simulink subsystem "Corrections"  (R2023b)
settings: Solver=VariableStepAuto  StartTime=0.0  StopTime=10.0  RelTol=1e-3
values from neighbouring files (symbols this model uses):
  c = obj.body_coeffs.Cnm.value    [SH_nav.m]
undefined symbols (not defined in the file or in its folder): Propagation, R_st, v_b, v_m, x_b, x_m
libraries: nav_lib x10, simulink x2, matrix_library x2, vrlib x1
settings Model: Creator=brent  LastModifiedBy=brent

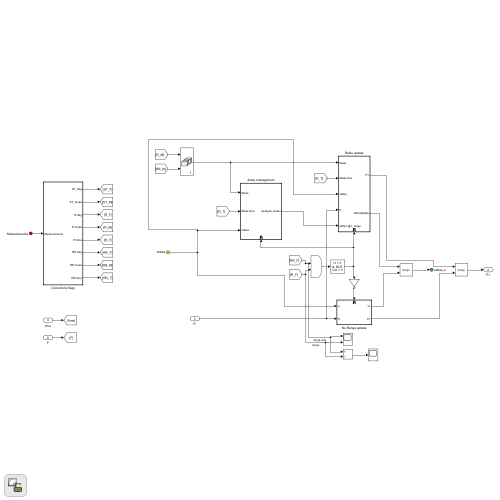
[thumbnail: Simulink's stored preview of the top-level diagram]
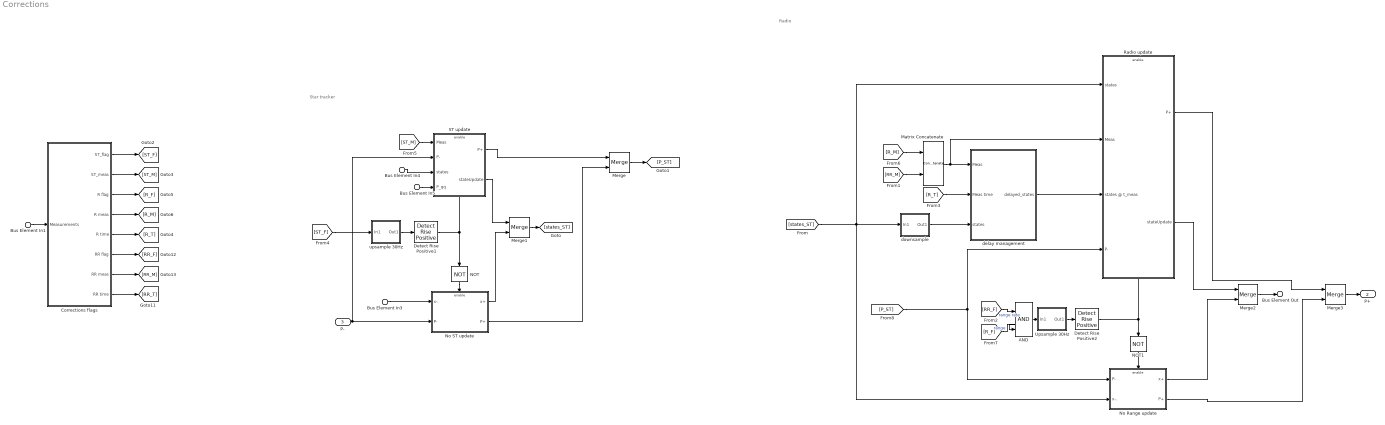
== system Corrections ==
  note: Radio
  note: Star tracker
  Bus Element In1 : Inport  PortName=Measurements
  Bus Element In5 : Inport  PortName=Measurements  Element=starTracker.P_qq
  Bus Element In3 : Inport  Port=2  PortName=states
  Bus Element In4 : Inport  Port=2  PortName=states
  P- : Inport  Port=3
  AND : Logic  IconShape=distinctive  AllPortsSameDT=off  OutDataTypeStr=boolean
  Corrections flags : Subsystem  TreatAsAtomicUnit=on  SystemSampleTime=1/Propagation.lf.value
  Detect Rise Positive1 : simulink/Logic and Bit Operations/Detect Rise Positive  vinit=0  OutDataTypeStr=boolean
  Detect Rise Positive2 : simulink/Logic and Bit Operations/Detect Rise Positive  vinit=0  OutDataTypeStr=boolean
  Matrix Concatenate : Concatenate  Mode=Multidimensional array
  Merge{,1..3} (4 alike) : Merge
  NOT : Logic  Operator=NOT  IconShape=distinctive  AllPortsSameDT=off  OutDataTypeStr=boolean
  NOT1 : Logic  Operator=NOT  IconShape=distinctive  AllPortsSameDT=off  OutDataTypeStr=boolean
  No Range update : Subsystem  TreatAsAtomicUnit=on
  No ST update : Subsystem  TreatAsAtomicUnit=on
  Radio update : Subsystem  TreatAsAtomicUnit=on
  ST update : Subsystem  TreatAsAtomicUnit=on
  Upsample 30Hz : Subsystem  TreatAsAtomicUnit=on  SystemSampleTime=1/Propagation.hf.value
  delay management : Subsystem  TreatAsAtomicUnit=on  SystemSampleTime=1/Propagation.lf.value
  downsample : Subsystem  TreatAsAtomicUnit=on  SystemSampleTime=1/Propagation.lf.value
  upsample 30Hz : Subsystem  TreatAsAtomicUnit=on  SystemSampleTime=1/Propagation.hf.value
  Bus Element Out : Outport  PortName=states_k
  P+ : Outport  Port=2
  wires:
  NOT1/1 -> No Range update/Enable
  No Range update/1(x+) -> Merge2/2
  Radio update/2(stateUpdate) -> Merge2/1
  Bus Element In1/1 -> Corrections flags/1(Measurements)
  Corrections flags/1(ST_flag) -> [ST_F]
  Corrections flags/2(ST_meas) -> [ST_M]
  Corrections flags/5(R time) -> [R_T]
  Corrections flags/4(R meas) -> [R_M]
  Corrections flags/3(R flag) -> [R_F]
  No Range update/2(P+) -> Merge3/2
  Radio update/1(P+) -> Merge3/1
  Corrections flags/6(RR flag) -> [RR_F]
  Corrections flags/7(RR meas) -> [RR_M]
  Corrections flags/8(RR time) -> [RR_T]
  [R_F] -> AND/2  "range"
  [RR_F] -> AND/1  "range rate"
  [RR_M] -> Matrix Concatenate/2
  [R_M] -> Matrix Concatenate/1
  Matrix Concatenate/1 -> delay management/1(Meas), Radio update/2(Meas)
  [R_T] -> delay management/2(Meas time)
  No ST update/1(x+) -> Merge1/2
  ST update/1(P+) -> Merge/1
  No ST update/2(P+) -> Merge/2
  Bus Element In3/1 -> No ST update/1(x-.)
  Detect Rise Positive1/1 -> NOT/1, ST update/Enable
  Bus Element In4/1 -> ST update/3(states)
  NOT/1 -> No ST update/Enable
  [ST_M] -> ST update/1(Meas)
  P-/1 -> ST update/2(P-), No ST update/2(P-)
  ST update/2(stateUpdate) -> Merge1/1
  upsample 30Hz/1(Out1) -> Detect Rise Positive1/1
  [states_ST] -> No Range update/2(x-.), downsample/1(In1), Radio update/1(states)
  AND/1 -> Upsample 30Hz/1(In1)
  Upsample 30Hz/1(Out1) -> Detect Rise Positive2/1
  [P_ST] -> Radio update/4(P-), No Range update/1(P-)
  downsample/1(Out1) -> delay management/3(states)
  Merge1/1 -> [states_ST]
  Merge/1 -> [P_ST]
  delay management/1(delayed_states) -> Radio update/3(states @ t_meas)
  Merge3/1 -> P+/1
  Merge2/1 -> Bus Element Out/1
  Bus Element In5/1 -> ST update/4(P_qq)
  Detect Rise Positive2/1 -> NOT1/1, Radio update/Enable
  [ST_F] -> upsample 30Hz/1(In1)

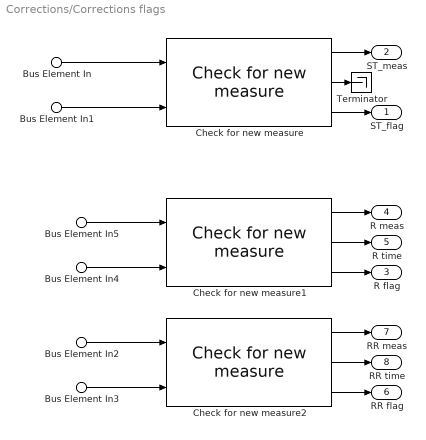
== system Corrections/Corrections flags ==
  Bus Element In5 : Inport  PortName=Measurements  Element=radio.range_PN
  Bus Element In2 : Inport  PortName=Measurements  Element=radio.range_rate
  Bus Element In4 : Inport  PortName=Measurements  Element=radio.range_timestamp
  Bus Element In3 : Inport  PortName=Measurements  Element=radio.range_rate_timestamp
  Bus Element In1 : Inport  PortName=Measurements  Element=starTracker.timestamp
  Bus Element In : Inport  PortName=Measurements  Element=starTracker.quaternion
  Check for new measure : nav_lib/Check for new measure  Ts=Propagation.lf.value
      settings: SourceProductName=Navigation library
  Check for new measure1 : nav_lib/Check for new measure  Ts=Inf
      settings: SourceProductName=Navigation library
  Check for new measure2 : nav_lib/Check for new measure  Ts=Inf
      settings: SourceProductName=Navigation library
  Terminator : Terminator
  ST_flag : Outport
  ST_meas : Outport  Port=2
  R flag : Outport  Port=3
  R meas : Outport  Port=4
  R time : Outport  Port=5
  RR flag : Outport  Port=6
  RR meas : Outport  Port=7
  RR time : Outport  Port=8
  wires:
  Check for new measure2/3 -> RR flag/1
  Check for new measure2/1 -> RR meas/1
  Check for new measure2/2 -> RR time/1
  Bus Element In2/1 -> Check for new measure2/1
  Bus Element In3/1 -> Check for new measure2/2
  Bus Element In4/1 -> Check for new measure1/2
  Bus Element In5/1 -> Check for new measure1/1
  Check for new measure1/2 -> R time/1
  Check for new measure1/1 -> R meas/1
  Check for new measure1/3 -> R flag/1
  Check for new measure/1 -> ST_meas/1
  Check for new measure/3 -> ST_flag/1
  Check for new measure/2 -> Terminator/1
  Bus Element In/1 -> Check for new measure/1
  Bus Element In1/1 -> Check for new measure/2

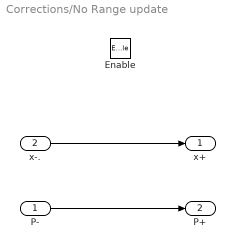
== system Corrections/No Range update ==
  P- : Inport
  x-. : Inport  Port=2
  Enable : EnablePort
  x+ : Outport
  P+ : Outport  Port=2
  wires:
  x-./1 -> x+/1
  P-/1 -> P+/1

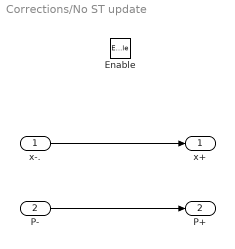
== system Corrections/No ST update ==
  x-. : Inport
  P- : Inport  Port=2
  Enable : EnablePort
  x+ : Outport
  P+ : Outport  Port=2
  wires:
  P-/1 -> P+/1
  x-./1 -> x+/1

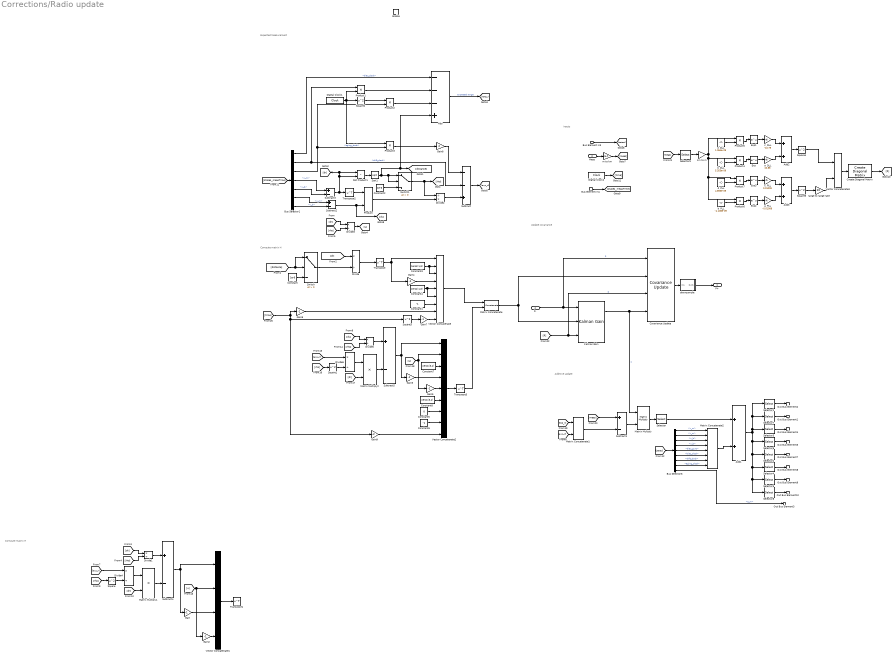
== system Corrections/Radio update ==
  note: Compute matrix H
  note: Additive update
  note: Update covariance
  note: Expected Measurement
  note: Compute matrix H
  note: Inputs
  Bus Element In3 : Inport  PortName=states
  Meas : Inport  Port=2
  Bus Element In1 : Inport  Port=3  PortName=states @ t_meas
  P- : Inport  Port=4
  Enable : EnablePort
  Add : Sum  Inputs=---+
  Add1 : Sum
  Add2 : Sum
  Add3 : Sum
  Bus Selector1 : BusSelector  OutputSignals=bias_clock,drift_clock,aging_clock,x_m,x_b,v_m,v_b
  Bus Selector6 : BusSelector  OutputSignals=x_m,v_m,x_b,v_b,bias_gyro,bias_clock,drift_clock,aging_clock,q_m
  Constant : Constant  Value=1e-6
  Constant1 : Constant  Value=-1  VectorParams1D=off
  Constant2 : Constant  Value=1e-6
  Constant3 : Constant  Value=zeros(1,3)  VectorParams1D=off
  Constant4 : Constant  Value=zeros(1,3)  VectorParams1D=off
  Constant5 : Constant  Value=0
  Constant6 : Constant  Value=-1
  Constant7 : Constant  Value=zeros(3,1)
  Constant8 : Constant  Value=zeros(3,1)
  Covariance Update : nav_lib/Covariance Update
      settings: SourceProductName=Navigation library
  Create Diagonal Matrix : matrix_library/Create Diagonal Matrix
      settings: LibrarySourceBlock=|
      | simulink/Matrix
      | Operations/Create Diagonal
      | Matrix
  Digital Clock1 : DigitalClock  SampleTime=-1
  Digital Clock2 : DigitalClock  SampleTime=-1
  Divide{,1,3..6} (6 alike) : Product  Inputs=*/
  Divide2 : Product  Inputs=/*
  Dot Product1 : DotProduct  OutDataTypeStr=Inherit: Inherit via internal rule
  Exp{,1..3} (4 alike) : Math
  Gain{,2..7} (7 alike) : Gain  Gain=-1
  Gain8 : Gain  Gain=2
  Gain9 : Gain  Gain=-2
  Kalman Gain : nav_lib/Kalman Gain
      settings: SourceProductName=Navigation library
  Matrix Concatenate : Concatenate  Mode=Multidimensional array
  Matrix Concatenate1 : Concatenate  Mode=Multidimensional array
  Matrix Concatenate2 : Concatenate  NumInputs=8  Mode=Multidimensional array
  Matrix Multiply : Product  Multiplication=Matrix(*)
  Matrix Multiply1 : Product
  Matrix Multiply2 : Product
  Product : Product  Multiplication=Matrix(*)
  Product{1..7} (7 alike) : Product
  Selector : Selector  NumberOfDimensions=2  InputPortWidth=3  IndexOptions=Index vector (dialog),Select all  Indices=[1:6 10:21],1  OutputSizes=1,1
  Selector1 : Selector  InputPortWidth=18  IndexOptions=Index vector (dialog)  Indices=1:3  OutputSizes=1
  Selector2 : Selector  InputPortWidth=18  IndexOptions=Index vector (dialog)  Indices=13:15  OutputSizes=1
  Selector3 : Selector  InputPortWidth=18  IndexOptions=Index vector (dialog)  Indices=7:9  OutputSizes=1
  Selector4 : Selector  InputPortWidth=18  IndexOptions=Index vector (dialog)  Indices=16  OutputSizes=1
  Selector5 : Selector  InputPortWidth=18  IndexOptions=Index vector (dialog)  Indices=17  OutputSizes=1
  Selector6 : Selector  InputPortWidth=18  IndexOptions=Index vector (dialog)  Indices=10:12  OutputSizes=1
  Selector7 : Selector  InputPortWidth=18  IndexOptions=Index vector (dialog)  Indices=4:6  OutputSizes=1
  Selector8 : Selector  InputPortWidth=18  IndexOptions=Index vector (dialog)  Indices=18  OutputSizes=1
  Selector9 : Selector  InputPortWidth=2  IndexOptions=Index vector (dialog)  Indices=1  OutputSizes=1
  Sqrt1 : Sqrt
  Square{,1..5} (6 alike) : Math  Operator=square
  Subtract : Sum  Inputs=--+
  Subtract{1..5} (5 alike) : Sum  Inputs=+-
  Switch : Switch  Criteria=u2 > Threshold  SaturateOnIntegerOverflow=off  InputSameDT=off
  Switch1 : Switch  Criteria=u2 > Threshold  SaturateOnIntegerOverflow=off  InputSameDT=off
  Transpose{,1..3} (4 alike) : Math  Operator=transpose
  Vector Concatenate : Concatenate  NumInputs=9  Mode=Multidimensional array  ConcatenateDimension=2
  Vector Concatenate1 : Concatenate  NumInputs=4  Mode=Multidimensional array
  Vector Concatenate2 : Concatenate  NumInputs=9  Mode=Multidimensional array
  Vector Concatenate3 : Concatenate
  a_DLL : Gain  Gain=10.88
  a_PLL : Gain  Gain=-0.01008
  b_DLL : Constant  Value=5.353e-09
  b_PLL : Constant  Value=-4.108e-09
  c_DLL : Gain  Gain=-10.79
  c_PLL : Gain  Gain=0.01009
  d_DLL : Constant  Value=1.064e-09
  d_PLL : Constant  Value=4.893e-09
  downsample : Subsystem  TreatAsAtomicUnit=on  SystemSampleTime=1/Propagation.lf.value
  km to m : Gain  Gain=1000
  m to km : Gain  Gain=1e-3
  range to range rate : Gain  Gain=20
  P+ : Outport
  Out Bus Element2 : Outport  Port=2  PortName=stateUpdate  Element=x_m
  Out Bus Element1 : Outport  Port=2  PortName=stateUpdate  Element=v_m
  Out Bus Element3 : Outport  Port=2  PortName=stateUpdate  Element=q_m
  Out Bus Element4 : Outport  Port=2  PortName=stateUpdate  Element=x_b
  Out Bus Element5 : Outport  Port=2  PortName=stateUpdate  Element=v_b
  Out Bus Element7 : Outport  Port=2  PortName=stateUpdate  Element=bias_gyro
  Out Bus Element8 : Outport  Port=2  PortName=stateUpdate  Element=bias_clock
  Out Bus Element9 : Outport  Port=2  PortName=stateUpdate  Element=drift_clock
  Out Bus Element10 : Outport  Port=2  PortName=stateUpdate  Element=aging_clock
  wires:
  range to range rate/1 -> Vector Concatenate3/2
  [R] -> Kalman Gain/3, Covariance Update/3  "R"
  Create Diagonal Matrix/1 -> [R]
  Vector Concatenate3/1 -> Create Diagonal Matrix/1
  Square4/1 -> Vector Concatenate3/1
  Square5/1 -> range to range rate/1
  Exp2/1 -> a_PLL/1
  Product6/1 -> Exp2/1
  b_PLL/1 -> Product6/2
  Exp3/1 -> c_PLL/1
  c_PLL/1 -> Add3/1
  Add3/1 -> Square5/1
  a_PLL/1 -> Add3/2
  d_PLL/1 -> Product7/2
  Product7/1 -> Exp3/1
  Add2/1 -> Square4/1
  c_DLL/1 -> Add2/1
  a_DLL/1 -> Add2/2
  Exp1/1 -> c_DLL/1
  Product5/1 -> Exp1/1
  d_DLL/1 -> Product5/2
  km to m/1 -> Product5/1, Product4/1, Product6/1, Product7/1
  Exp/1 -> a_DLL/1
  Product4/1 -> Exp/1
  b_DLL/1 -> Product4/2
  Selector9/1 -> km to m/1
  [meas] -> Selector9/1
  Subtract1/1 -> Matrix Multiply/2
  downsample/1(Out1) -> P+/1
  Selector8/1 -> Out Bus Element10/1
  Selector5/1 -> Out Bus Element9/1
  Selector4/1 -> Out Bus Element8/1
  Selector2/1 -> Out Bus Element7/1
  Selector6/1 -> Out Bus Element5/1
  Selector3/1 -> Out Bus Element4/1
  Bus Selector6/9 -> Out Bus Element3/1  "<q_m>"
  Selector7/1 -> Out Bus Element1/1
  Selector1/1 -> Out Bus Element2/1
  Bus Selector6/8 -> Matrix Concatenate2/8  "<aging_clock>"
  Bus Selector6/7 -> Matrix Concatenate2/7  "<drift_clock>"
  Bus Selector6/6 -> Matrix Concatenate2/6  "<bias_clock>"
  Bus Selector6/5 -> Matrix Concatenate2/5  "<bias_gyro>"
  Selector/1 -> Add1/1
  Add1/1 -> Selector6/1, Selector2/1, Selector4/1, Selector5/1, Selector8/1, Selector7/1, Selector1/1, Selector3/1
  Constant8/1 -> Vector Concatenate2/6
  Constant5/1 -> Vector Concatenate2/7
  Constant6/1 -> Vector Concatenate2/8
  Gain9/1 -> Vector Concatenate2/9
  Gain5/1 -> Vector Concatenate2/5
  Gain3/1 -> Vector Concatenate2/4
  Constant7/1 -> Vector Concatenate2/3
  Gain7/1 -> Vector Concatenate/9
  Constant1/1 -> Vector Concatenate/7
  Constant4/1 -> Vector Concatenate/5, Vector Concatenate/6
  Gain4/1 -> Vector Concatenate/4
  Gain6/1 -> Vector Concatenate/8
  [states_measTime] -> Bus Selector1/1
  Bus Element In1/1 -> [states_measTime]
  Digital Clock2/1 -> [time]
  [meas] -> Subtract1/1
  m to km/1 -> [meas]
  Meas/1 -> m to km/1
  Gain8/1 -> Subtract/1
  Product3/1 -> Gain8/1
  Divide2/1 -> Subtract/3
  Product2/1 -> Add/3
  Square2/1 -> Product2/1
  Bus Selector1/3 -> Product2/2, Product3/2  "<aging_clock>"
  Square3/1 -> Gain7/1
  [time] -> Gain6/1, Square3/1, Gain9/1
  Subtract/1 -> [exp_rr]
  Product1/1 -> Add/2
  Bus Selector1/2 -> Product1/1, Subtract/2  "<drift_clock>"
  Digital Clock1/1 -> Square2/1, Product1/2, Product3/1
  Bus Selector1/1 -> Add/1  "<bias_clock>"
  [exp_r] -> Matrix Concatenate1/1
  [exp_rr] -> Matrix Concatenate1/2
  Vector Concatenate/1 -> Matrix Concatenate/1
  Transpose3/1 -> Matrix Concatenate/2
  Matrix Concatenate/1 -> Covariance Update/2, Kalman Gain/2
  [rho] -> Square1/1
  Subtract5/1 -> Vector Concatenate2/1, Gain3/1
  Divide6/1 -> Matrix Multiply2/1
  Divide5/1 -> Subtract5/1
  Square1/1 -> Divide6/2
  [exp_rr] -> Divide6/1
  [dr] -> Matrix Multiply2/2
  [dv] -> Divide5/1
  [rho] -> Divide5/2
  Matrix Multiply2/1 -> Subtract5/2
  Vector Concatenate2/1 -> Transpose3/1
  [u] -> Vector Concatenate2/2, Gain5/1
  Switch1/1 -> [rho], Divide2/1
  Subtract4/1 -> Vector Concatenate1/1, Gain/1
  Bus Selector1/7 -> Subtract2/2  "<v_b>"
  Divide3/1 -> [u]
  Divide1/1 -> Subtract4/1
  Bus Selector1/4 -> Subtract3/1  "<x_m>"
  Dot Product1/1 -> Sqrt1/1
  Sqrt1/1 -> [distance], Add/4, Switch1/1, Switch1/2
  Subtract3/1 -> Transpose2/1, Dot Product1/2, [dr], Dot Product1/1
  Constant2/1 -> Switch1/3
  [dr] -> Divide3/1
  [rho] -> Square/1
  Product/1 -> Divide2/2
  Bus Selector1/5 -> Subtract3/2  "<x_b>"
  [exp_rr] -> Divide4/1
  Gain2/1 -> Vector Concatenate1/4
  Square/1 -> Divide4/2
  [rho] -> Divide3/2
  Divide4/1 -> Matrix Multiply1/1
  [dr] -> Matrix Multiply1/2
  [dv] -> Divide1/1
  Subtract2/1 -> Product/2, [dv]
  [rho] -> Divide1/2
  Vector Concatenate1/1 -> Transpose1/1
  Matrix Multiply1/1 -> Subtract4/2
  Transpose2/1 -> Product/1
  Gain/1 -> Vector Concatenate1/3
  [u] -> Gain2/1, Vector Concatenate1/2
  Bus Selector1/6 -> Subtract2/1  "<v_m>"
  Transpose/1 -> Vector Concatenate/1, Gain4/1
  Bus Selector6/4 -> Matrix Concatenate2/4  "<v_b>"
  Bus Selector6/2 -> Matrix Concatenate2/2  "<v_m>"
  Constant3/1 -> Vector Concatenate/2, Vector Concatenate/3
  Covariance Update/1 -> downsample/1(In1)
  Bus Selector6/3 -> Matrix Concatenate2/3  "<x_b>"
  [dr] -> Divide/1
  Kalman Gain/1 -> Matrix Multiply/1, Covariance Update/4  "K"
  P-/1 -> Kalman Gain/1, Covariance Update/1  "P"
  Matrix Concatenate1/1 -> Subtract1/2
  Bus Selector6/1 -> Matrix Concatenate2/1  "<x_m>"
  Matrix Concatenate2/1 -> Add1/2
  [states] -> Bus Selector6/1
  Matrix Multiply/1 -> Selector/1
  Divide/1 -> Transpose/1
  Switch/1 -> Divide/2
  Constant/1 -> Switch/3
  [distance] -> Switch/2, Switch/1
  Add/1 -> [exp_r]  "expected range"
  Bus Element In3/1 -> [states]

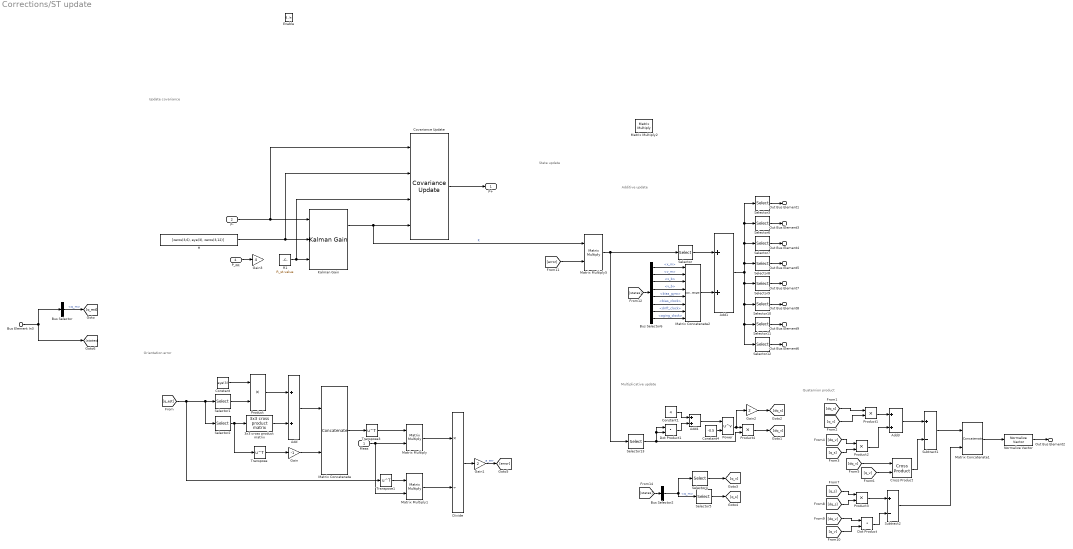
== system Corrections/ST update ==
  note: Orientation error
  note: Update covariance
  note: State update
  note: Additive update
  note: Multiplicative update
  note: Quaternion product
  Meas : Inport
  P- : Inport  Port=2
  Bus Element In3 : Inport  Port=3  PortName=states
  P_qq : Inport  Port=4
  Enable : EnablePort
  3x3 cross product matrix : nav_lib/3x3 cross product matrix
      settings: SourceProductName=Navigation library
  Add{,1,3..4} (4 alike) : Sum
  Bus Selector : BusSelector  OutputSignals=q_m
  Bus Selector2 : BusSelector  OutputSignals=q_m
  Bus Selector6 : BusSelector  OutputSignals=x_m,v_m,x_b,v_b,bias_gyro,bias_clock,drift_clock,aging_clock
  Constant : Constant  Value=eye(3)
  Constant1 : Constant  Value=4
  Constant4 : Constant  Value=-0.5
  Covariance Update : nav_lib/Covariance Update
      settings: SourceProductName=Navigation library
  Cross Product : matrix_library/Cross Product
  Divide : Product  Inputs=*/
  Dot Product : DotProduct  OutDataTypeStr=Inherit: Inherit via internal rule
  Dot Product1 : DotProduct  OutDataTypeStr=Inherit: Inherit via internal rule
  Gain : Gain  Gain=-1
  Gain1 : Gain  Gain=2
  Gain2 : Gain  Gain=2
  Gain3 : Gain  Gain=4
  H : Constant  Value=[zeros(3,6), eye(3), zeros(3,12)]
  Kalman Gain : nav_lib/Kalman Gain
      settings: SourceProductName=Navigation library
  Matrix Concatenate : Concatenate  Mode=Multidimensional array
  Matrix Concatenate1 : Concatenate  Mode=Multidimensional array
  Matrix Concatenate2 : Concatenate  NumInputs=8  Mode=Multidimensional array
  Matrix Multiply{,1..2,5} (4 alike) : Product  Multiplication=Matrix(*)
  Normalize Vector : vrlib/Utilities/Normalize Vector  maxzero=0
  Power : Math  Operator=pow
  Product{,1..4} (5 alike) : Product
  R1 : Constant  Value=R_st.value
  Selector : Selector  InputPortWidth=21  IndexOptions=Index vector (dialog)  Indices=[1:6 10:21]  OutputSizes=1
  Selector1 : Selector  InputPortWidth=4  IndexOptions=Index vector (dialog)  Indices=4  OutputSizes=1
  Selector10 : Selector  InputPortWidth=18  IndexOptions=Index vector (dialog)  Indices=16  OutputSizes=1
  Selector11 : Selector  InputPortWidth=18  IndexOptions=Index vector (dialog)  Indices=17  OutputSizes=1
  Selector12 : Selector  InputPortWidth=18  IndexOptions=Index vector (dialog)  Indices=18  OutputSizes=1
  Selector13 : Selector  InputPortWidth=21  IndexOptions=Index vector (dialog)  Indices=7:9  OutputSizes=1
  Selector2 : Selector  InputPortWidth=4  IndexOptions=Index vector (dialog)  Indices=1:3  OutputSizes=1
  Selector3 : Selector  InputPortWidth=18  IndexOptions=Index vector (dialog)  Indices=1:3  OutputSizes=1
  Selector4 : Selector  InputPortWidth=4  IndexOptions=Index vector (dialog)  Indices=1:3  OutputSizes=1
  Selector5 : Selector  InputPortWidth=4  IndexOptions=Index vector (dialog)  Indices=4  OutputSizes=1
  Selector6 : Selector  InputPortWidth=18  IndexOptions=Index vector (dialog)  Indices=4:6  OutputSizes=1
  Selector7 : Selector  InputPortWidth=18  IndexOptions=Index vector (dialog)  Indices=7:9  OutputSizes=1
  Selector8 : Selector  InputPortWidth=18  IndexOptions=Index vector (dialog)  Indices=10:12  OutputSizes=1
  Selector9 : Selector  InputPortWidth=18  IndexOptions=Index vector (dialog)  Indices=13:15  OutputSizes=1
  Subtract1 : Sum  Inputs=+-
  Subtract2 : Sum  Inputs=+-
  Transpose : Math  Operator=transpose
  Transpose1 : Math  Operator=transpose
  Transpose3 : Math  Operator=transpose
  P+ : Outport
  Out Bus Element1 : Outport  Port=2  PortName=stateUpdate  Element=x_m
  Out Bus Element3 : Outport  Port=2  PortName=stateUpdate  Element=v_m
  Out Bus Element2 : Outport  Port=2  PortName=stateUpdate  Element=q_m
  Out Bus Element4 : Outport  Port=2  PortName=stateUpdate  Element=x_b
  Out Bus Element5 : Outport  Port=2  PortName=stateUpdate  Element=v_b
  Out Bus Element7 : Outport  Port=2  PortName=stateUpdate  Element=bias_gyro
  Out Bus Element8 : Outport  Port=2  PortName=stateUpdate  Element=bias_clock
  Out Bus Element9 : Outport  Port=2  PortName=stateUpdate  Element=drift_clock
  Out Bus Element6 : Outport  Port=2  PortName=stateUpdate  Element=aging_clock
  wires:
  R1/1 -> Kalman Gain/3, Covariance Update/3
  P_qq/1 -> Gain3/1
  Covariance Update/1 -> P+/1
  Selector12/1 -> Out Bus Element6/1
  Selector11/1 -> Out Bus Element9/1
  Selector10/1 -> Out Bus Element8/1
  Bus Selector6/8 -> Matrix Concatenate2/8  "<aging_clock>"
  Bus Selector6/7 -> Matrix Concatenate2/7  "<drift_clock>"
  Bus Selector6/6 -> Matrix Concatenate2/6  "<bias_clock>"
  Bus Selector6/5 -> Matrix Concatenate2/5  "<bias_gyro>"
  Bus Selector6/1 -> Matrix Concatenate2/1  "<x_m>"
  Bus Selector6/2 -> Matrix Concatenate2/2  "<v_m>"
  Bus Selector6/3 -> Matrix Concatenate2/3  "<x_b>"
  Bus Selector6/4 -> Matrix Concatenate2/4  "<v_b>"
  [states] -> Bus Selector2/1
  Selector9/1 -> Out Bus Element7/1
  Selector8/1 -> Out Bus Element5/1
  Selector7/1 -> Out Bus Element4/1
  Selector6/1 -> Out Bus Element3/1
  Selector3/1 -> Out Bus Element1/1
  Add1/1 -> Selector11/1, Selector12/1, Selector10/1, Selector9/1, Selector3/1, Selector6/1, Selector7/1, Selector8/1
  Matrix Concatenate2/1 -> Add1/2
  Selector/1 -> Add1/1
  [states] -> Bus Selector6/1
  Bus Element In3/1 -> Bus Selector/1, [states]
  Bus Selector/1 -> [q_est]  "<q_m>"
  [error] -> Matrix Multiply5/2
  Gain1/1 -> [error]  "a_err"
  H/1 -> Kalman Gain/2, Covariance Update/2
  P-/1 -> Kalman Gain/1, Covariance Update/1
  Product4/1 -> [dq_v]
  Gain2/1 -> [dq_s]
  Selector4/1 -> [q_v]
  Selector5/1 -> [q_s]
  Power/1 -> Product4/1, Gain2/1
  Constant4/1 -> Power/2
  Add4/1 -> Power/1
  Dot Product1/1 -> Add4/2
  Constant1/1 -> Add4/1
  Kalman Gain/1 -> Covariance Update/4, Matrix Multiply5/1  "K"
  Normalize Vector/1 -> Out Bus Element2/1
  Matrix Concatenate1/1 -> Normalize Vector/1
  Subtract2/1 -> Matrix Concatenate1/2
  Product3/1 -> Subtract2/1
  Dot Product/1 -> Subtract2/2
  [q_v] -> Dot Product/2
  [dq_v] -> Dot Product/1
  [q_s] -> Product3/1
  [dq_s] -> Product3/2
  Subtract1/1 -> Matrix Concatenate1/1
  Cross Product/1 -> Subtract1/2
  [q_v] -> Cross Product/2
  [dq_v] -> Cross Product/1
  Add3/1 -> Subtract1/1
  Product2/1 -> Add3/2
  [dq_v] -> Product2/1
  [q_s] -> Product2/2
  Product1/1 -> Add3/1
  [q_v] -> Product1/2
  [dq_s] -> Product1/1
  Bus Selector2/1 -> Selector5/1, Selector4/1  "<q_m>"
  Selector13/1 -> Product4/2, Dot Product1/2, Dot Product1/1
  Matrix Multiply5/1 -> Selector/1, Selector13/1
  Transpose3/1 -> Matrix Multiply/1
  Divide/1 -> Gain1/1
  Matrix Multiply1/1 -> Divide/2
  Matrix Multiply/1 -> Divide/1
  Transpose1/1 -> Matrix Multiply1/1
  Meas/1 -> Matrix Multiply1/2, Matrix Multiply/2
  Matrix Concatenate/1 -> Transpose3/1
  Add/1 -> Matrix Concatenate/1
  Gain/1 -> Matrix Concatenate/2
  Transpose/1 -> Gain/1
  Product/1 -> Add/1
  3x3 cross product matrix/1 -> Add/2
  Selector2/1 -> 3x3 cross product matrix/1, Transpose/1
  Constant/1 -> Product/1
  Selector1/1 -> Product/2
  [q_est] -> Selector1/1, Selector2/1, Transpose1/1

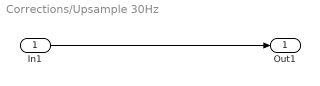
== system Corrections/Upsample 30Hz ==
  In1 : Inport
  Out1 : Outport
  wires:
  In1/1 -> Out1/1

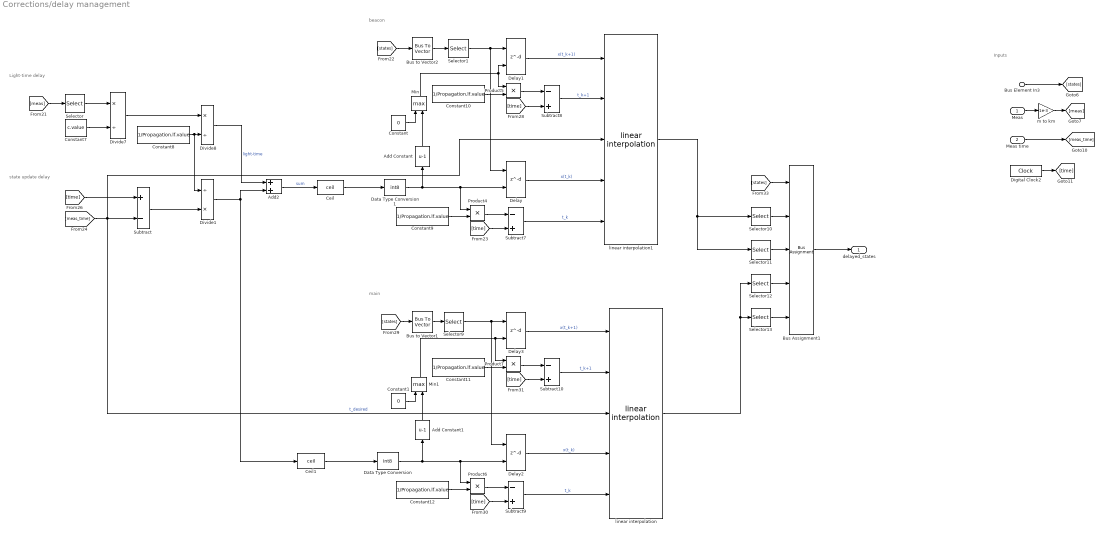
== system Corrections/delay management ==
  note: Inputs
  note: Light-time delay
  note: state update delay
  note: main
  note: beacon
  Meas : Inport
  Meas time : Inport  Port=2
  Bus Element In3 : Inport  Port=3  PortName=states
  Add Constant : Bias  Bias=-1  SaturateOnIntegerOverflow=off
  Add Constant1 : Bias  Bias=-1  SaturateOnIntegerOverflow=off
  Add2 : Sum
  Bus Assignment1 : BusAssignment  AssignedSignals=x_b,v_b,x_m,v_m
  Bus to Vector1 : BusToVector
  Bus to Vector2 : BusToVector
  Ceil : Rounding  Operator=ceil
  Ceil1 : Rounding  Operator=ceil
  Constant : Constant  Value=0
  Constant1 : Constant  Value=0
  Constant{8..12} (5 alike) : Constant  Value=1/Propagation.lf.value
  Constant7 : Constant  Value=c.value
  Data Type Conversion : DataTypeConversion  OutDataTypeStr=int8  SaturateOnIntegerOverflow=off  RndMeth=Floor
  Data Type Conversion1 : DataTypeConversion  OutDataTypeStr=int8  SaturateOnIntegerOverflow=off  RndMeth=Floor
  Delay : Delay  DelayLengthSource=Input port  DelayLengthUpperLimit=4
      settings: InputPortMap=u0,p1
  Delay1 : Delay  DelayLengthSource=Input port  DelayLengthUpperLimit=4  InitialCondition=0  UseCircularBuffer=on
      settings: InputPortMap=u0,p1
  Delay2 : Delay  DelayLengthSource=Input port  DelayLengthUpperLimit=4
      settings: InputPortMap=u0,p1
  Delay3 : Delay  DelayLengthSource=Input port  DelayLengthUpperLimit=4
      settings: InputPortMap=u0,p1
  Digital Clock2 : DigitalClock  SampleTime=-1
  Divide1 : Product  Inputs=/*
  Divide7 : Product  Inputs=*/
  Divide8 : Product  Inputs=*/
  Min : MinMax  Function=max  Inputs=2
  Min1 : MinMax  Function=max  Inputs=2
  Product{4..7} (4 alike) : Product
  Selector : Selector  NumberOfDimensions=2  InputPortWidth=3  IndexOptions=Index vector (dialog),Index vector (dialog)  Indices=1,1  OutputSizes=1,1
  Selector1 : Selector  InputPortWidth=22  IndexOptions=Index vector (dialog)  Indices=11:16  OutputSizes=1
  Selector10 : Selector  InputPortWidth=6  IndexOptions=Index vector (dialog)  Indices=1:3  OutputSizes=1
  Selector11 : Selector  InputPortWidth=6  IndexOptions=Index vector (dialog)  Indices=4:6  OutputSizes=1
  Selector12 : Selector  InputPortWidth=6  IndexOptions=Index vector (dialog)  Indices=1:3  OutputSizes=1
  Selector13 : Selector  InputPortWidth=6  IndexOptions=Index vector (dialog)  Indices=4:6  OutputSizes=1
  Selector9 : Selector  InputPortWidth=22  IndexOptions=Index vector (dialog)  Indices=1:6  OutputSizes=1
  Subtract : Sum  Inputs=+-
  Subtract{7..10} (4 alike) : Sum  Inputs=-+
  linear interpolation : nav_lib/linear interpolation
      settings: SourceProductName=Navigation library
  linear interpolation1 : nav_lib/linear interpolation
      settings: SourceProductName=Navigation library
  m to km : Gain  Gain=1e-3
  delayed_states : Outport
  wires:
  Divide1/1 -> Ceil1/1, Add2/2
  linear interpolation/1 -> Selector13/1, Selector12/1
  Subtract/1 -> Divide1/2
  Data Type Conversion1/1 -> Add Constant/1, Delay/2, Product4/1
  Data Type Conversion/1 -> Add Constant1/1, Delay2/2, Product6/1
  Constant1/1 -> Min1/1
  Add Constant1/1 -> Min1/2
  Min1/1 -> Product7/1, Delay3/2
  Constant/1 -> Min/1
  Add Constant/1 -> Min/2
  Min/1 -> Delay1/2, Product5/1
  Bus to Vector2/1 -> Selector1/1
  Selector1/1 -> Delay1/1, Delay/1
  Meas/1 -> m to km/1
  Bus Element In3/1 -> [states]
  Meas time/1 -> [meas_time]
  m to km/1 -> [meas]
  Digital Clock2/1 -> [time]
  Divide8/1 -> Add2/1  "light-time"
  Selector10/1 -> Bus Assignment1/2
  Selector/1 -> Divide7/1
  [states] -> Bus to Vector2/1
  Constant12/1 -> Product6/2
  linear interpolation1/1 -> Selector10/1, Selector11/1
  [meas_time] -> Subtract/2, linear interpolation/3, linear interpolation1/3  "t_desired"
  Product7/1 -> Subtract10/1
  [states] -> Bus to Vector1/1
  Ceil/1 -> Data Type Conversion1/1
  Add2/1 -> Ceil/1  "sum"
  Bus Assignment1/1 -> delayed_states/1
  Bus to Vector1/1 -> Selector9/1
  Constant9/1 -> Product4/2
  [time] -> Subtract10/2
  Ceil1/1 -> Data Type Conversion/1
  [time] -> Subtract/1
  Delay3/1 -> linear interpolation/1  "x(t_k+1)"
  Delay1/1 -> linear interpolation1/1  "x(t_k+1)"
  Subtract8/1 -> linear interpolation1/2  "t_k+1"
  Constant7/1 -> Divide7/2
  Constant8/1 -> Divide8/2, Divide1/1
  Constant11/1 -> Product7/2
  Product4/1 -> Subtract7/1
  Selector11/1 -> Bus Assignment1/3
  [time] -> Subtract8/2
  Product5/1 -> Subtract8/1
  Constant10/1 -> Product5/2
  [meas] -> Selector/1
  [time] -> Subtract9/2
  Subtract10/1 -> linear interpolation/2  "t_k+1"
  Selector9/1 -> Delay3/1, Delay2/1
  Subtract9/1 -> linear interpolation/5  "t_k"
  Delay2/1 -> linear interpolation/4  "x(t_k)"
  Product6/1 -> Subtract9/1
  Subtract7/1 -> linear interpolation1/5  "t_k"
  Selector12/1 -> Bus Assignment1/4
  [states] -> Bus Assignment1/1
  Divide7/1 -> Divide8/1
  [time] -> Subtract7/2
  Delay/1 -> linear interpolation1/4  "x(t_k)"
  Selector13/1 -> Bus Assignment1/5

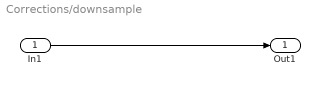
== system Corrections/downsample ==
  In1 : Inport
  Out1 : Outport
  wires:
  In1/1 -> Out1/1

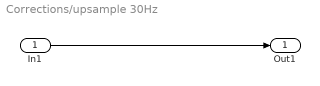
== system Corrections/upsample 30Hz ==
  In1 : Inport
  Out1 : Outport
  wires:
  In1/1 -> Out1/1

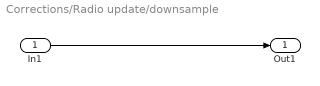
== system Corrections/Radio update/downsample ==
  In1 : Inport
  Out1 : Outport
  wires:
  In1/1 -> Out1/1
